simulink model "HLSDem_CalcState"  (R2016b)
settings: configuration reference "CodeGenConfigSet" (kept outside this file)
values from neighbouring files (symbols this model uses):
  EISGov_nOfsPreCtlActvFall_C = Calibration.Parameter    [init_HLSDem_CalcState.m]
  EISGov_nOfsPreCtlActvFall_CUR = Calibration.Parameter    [init_HLSDem_CalcState.m]
  EISGov_nOfsPreCtlActvFall_CURX = Calibration.Parameter    [init_HLSDem_CalcState.m]
  EISGov_nOfsPreCtlINActvFall_C = Calibration.Parameter    [init_HLSDem_CalcState.m]
  EISGov_nOfsPreCtlPrepFall_C = Calibration.Parameter    [init_HLSDem_CalcState.m]
  EISGov_nPreCtlPrepFalloffset_C = Calibration.Parameter    [init_HLSDem_CalcState.m]
  HLSDem_facGripPredef_CUR = Calibration.Parameter    [init_HLSDem_CalcState.m]
  HLSDem_facGripPredef_CURX = Calibration.Parameter    [init_HLSDem_CalcState.m]
  HLSDem_facNoGripPredef_CUR = Calibration.Parameter    [init_HLSDem_CalcState.m]
  HLSDem_facNoGripPredef_CURX = Calibration.Parameter    [init_HLSDem_CalcState.m]
  HLSDem_GripPredef_CUR = Calibration.Parameter    [init_HLSDem_CalcState.m]
  HLSDem_GripPredef_CURX = Calibration.Parameter    [init_HLSDem_CalcState.m]
  HLSDem_nOfsPredef_C = Calibration.Parameter    [init_HLSDem_CalcState.m]
  HLSDem_nOfsUndrBrk_C = Calibration.Parameter    [init_HLSDem_CalcState.m]
  HLSDem_NoGripPredef_C = Calibration.Parameter    [init_HLSDem_CalcState.m]
  HLSDem_numTempSelConv_C = Calibration.Parameter    [init_HLSDem_CalcState.m]
  HLSDem_rAPPThresFrzI_C = Calibration.Parameter    [init_HLSDem_CalcState.m]
  HLSDem_rAPPThresTrqDem_C = Calibration.Parameter    [init_HLSDem_CalcState.m]
  HLSDem_rGripUndrBrkThres_C = Calibration.Parameter    [init_HLSDem_CalcState.m]
  HLSDem_rNoGripThres_C = Calibration.Parameter    [init_HLSDem_CalcState.m]
  HLSDem_stIFrzInhib_C = Calibration.Parameter    [init_HLSDem_CalcState.m]
  HLSDem_swtAPPFrzI_C = Calibration.Parameter    [init_HLSDem_CalcState.m]
  HLSDem_swtAPPTrqDem_C = Calibration.Parameter    [init_HLSDem_CalcState.m]
  HLSDem_swtPredef_C = Calibration.Parameter    [init_HLSDem_CalcState.m]
  HLSDem_trqReqStrt_CUR = Calibration.Parameter    [init_HLSDem_CalcState.m]
  HLSDem_trqReqStrt_CURX = Calibration.Parameter    [init_HLSDem_CalcState.m]
  HLSDem_vThresUndrBrk_C = Calibration.Parameter    [init_HLSDem_CalcState.m]
  LIGov_nOffsetPreCtltrqDem_C = Calibration.Parameter    [init_HLSDem_CalcState.m]
undefined symbols (not defined in the file or in its folder): EISGov_num_conv, EngState_conv, PT_TraType_State_conv, Switch_conv
libraries: simulink x35, CXLib x2
settings Model: Creator=Administrator  LastModifiedBy=xuxingpei
settings ConfigSetRef: SourceLocation=Base Workspace

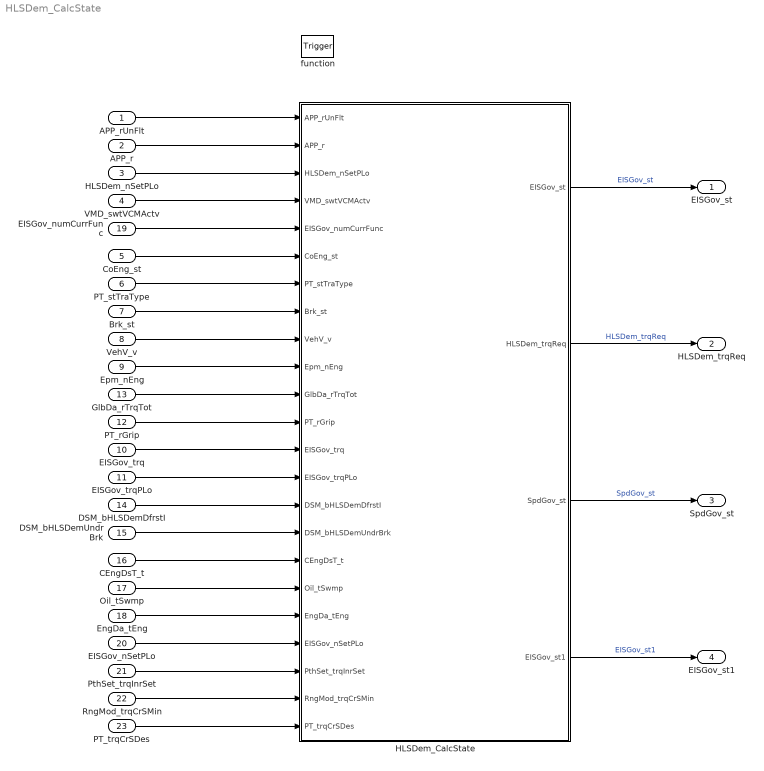
== system HLSDem_CalcState ==
  APP_rUnFlt : Inport  Tag=%  Description=Unfiltered APP value  OutMin=0  OutMax=100  OutDataTypeStr=Accpedal_rate
  APP_r : Inport  Tag=%  Description=Acceleration pedal sensor 1 value after fault handling  Port=2  OutMin=0  OutMax=100  OutDataTypeStr=Accpedal_rate
  HLSDem_nSetPLo : Inport  Tag=rpm  Description=Minimum engine speed of HLSDem  Port=3  OutMin=0  OutMax=6000  OutDataTypeStr=EngSpeed_rpm
  VMD_swtVCMActv : Inport  Description=Application parameter which Indicates whether Vehicle Control Mode(VCM) is enabled or disabled  Port=4  OutDataTypeStr=Enum: Switch_conv
  CoEng_st : Inport  Description=Engine coordinator state  Port=5  OutDataTypeStr=Enum: EngState_conv
  PT_stTraType : Inport  Description=Current transmission type  Port=6  OutDataTypeStr=Enum: PT_TraType_State_conv
  Brk_st : Inport  Description=Brake switch state  Port=7  OutMin=0  OutMax=255  OutDataTypeStr=State_uint8
  VehV_v : Inport  Tag=km/h  Description=Vehicle speed  Port=8  OutMin=0  OutMax=250  OutDataTypeStr=VehSpeed_km_h
  Epm_nEng : Inport  Tag=rpm  Description=Engine speed  Port=9  OutMin=0  OutMax=6000  OutDataTypeStr=EngSpeed_rpm
  EISGov_trq : Inport  Tag=Nm  Description=Resulted output torque of EISGov controller  Port=10  OutMin=-3276.8  OutMax=3276.7  OutDataTypeStr=Trq_Nm
  EISGov_trqPLo : Inport  Tag=Nm  Description=P-component of the lower path  Port=11  OutMin=-3276.8  OutMax=3276.7  OutDataTypeStr=Trq_Nm
  PT_rGrip : Inport  Description=Analogue value for the grip states  Port=12  OutMin=-300  OutMax=300  OutDataTypeStr=Prc_Fact100
  GlbDa_rTrqTot : Inport  Description=total ratio of the power train inclusive the differential and the converter torque ratio  Port=13  OutMin=-327  OutMax=327  OutDataTypeStr=TransRatio
  DSM_bHLSDemDfrstI : Inport  Description=Status of Fid_HLSDemDfrstI  Port=14  OutMin=0  OutMax=1  OutDataTypeStr=boolean
  DSM_bHLSDemUndrBrk : Inport  Description=Status of FId_HLSDemUndrBrk  Port=15  OutMin=0  OutMax=1  OutDataTypeStr=boolean
  CEngDsT_t : Inport  Tag=deg  Description=engine coolant temperature after filter  Port=16  OutMin=-200  OutMax=200  OutDataTypeStr=Temp_deg
  Oil_tSwmp : Inport  Tag=deg  Description=Oil temperature in oil sump  Port=17  OutMin=-50  OutMax=200  OutDataTypeStr=Temp_deg
  EngDa_tEng : Inport  Tag=deg  Description=Engine temperature  Port=18  OutMin=-1000  OutMax=1000  OutDataTypeStr=Temp_deg
  EISGov_numCurrFunc : Inport  Description=Identification name / number of the currently active EISGov client, which determines the current controller parameters  Port=19  OutDataTypeStr=Enum: EISGov_num_conv
  EISGov_nSetPLo : Inport  Tag=rpm  Description=Lower limit of the speed interval (set point speed) of the EISGov  Port=20  OutMin=0  OutMax=6000  OutDataTypeStr=EngSpeed_rpm
  PthSet_trqInrSet : Inport  Tag=Nm  Description=Inner torque set value after monitoring limitation  Port=21  OutMin=-3000  OutMax=3276.7  OutDataTypeStr=Trq_Nm
  RngMod_trqCrSMin : Inport  Tag=Nm  Description=minimal crankshaft torque  Port=22  OutMin=-3276.8  OutMax=3276.7  OutDataTypeStr=Trq_Nm
  PT_trqCrSDes : Inport  Tag=Nm  Description=Application parameter for requested propulsion torque to engine(crankshaft torque)  Port=23  OutMin=-3000  OutMax=3000  OutDataTypeStr=Trq_Nm
  function : TriggerPort  TriggerType=function-call  VariantControl=Variant
  HLSDem_CalcState : Subsystem
  EISGov_st : Outport  Description=Status information of EISGov and its clients  OutMin=0  OutMax=2147483648  OutDataTypeStr=State_uint32
  HLSDem_trqReq : Outport  Tag=Nm  Description=Requested initialisation torque to engine speed governor (with reference to the output)  Port=2  OutMin=-3000  OutMax=3000  OutDataTypeStr=Trq_Nm
  SpdGov_st : Outport  Description=status speed control SpdGov  Port=3  OutMin=0  OutMax=65535  OutDataTypeStr=State_uint16
  EISGov_st1 : Outport  Description=Status information of HLSDem client  Port=4  OutMin=0  OutMax=2147483648  OutDataTypeStr=State_uint32
  wires:
  PT_rGrip/1 -> HLSDem_CalcState/12(PT_rGrip)
  Epm_nEng/1 -> HLSDem_CalcState/10(Epm_nEng)
  APP_rUnFlt/1 -> HLSDem_CalcState/1(APP_rUnFlt)
  APP_r/1 -> HLSDem_CalcState/2(APP_r)
  VehV_v/1 -> HLSDem_CalcState/9(VehV_v)
  EISGov_numCurrFunc/1 -> HLSDem_CalcState/5(EISGov_numCurrFunc)
  PT_stTraType/1 -> HLSDem_CalcState/7(PT_stTraType)
  Brk_st/1 -> HLSDem_CalcState/8(Brk_st)
  CoEng_st/1 -> HLSDem_CalcState/6(CoEng_st)
  VMD_swtVCMActv/1 -> HLSDem_CalcState/4(VMD_swtVCMActv)
  EISGov_trq/1 -> HLSDem_CalcState/13(EISGov_trq)
  HLSDem_nSetPLo/1 -> HLSDem_CalcState/3(HLSDem_nSetPLo)
  EISGov_trqPLo/1 -> HLSDem_CalcState/14(EISGov_trqPLo)
  DSM_bHLSDemDfrstI/1 -> HLSDem_CalcState/15(DSM_bHLSDemDfrstI)
  DSM_bHLSDemUndrBrk/1 -> HLSDem_CalcState/16(DSM_bHLSDemUndrBrk)
  GlbDa_rTrqTot/1 -> HLSDem_CalcState/11(GlbDa_rTrqTot)
  HLSDem_CalcState/1(EISGov_st) -> EISGov_st/1  "EISGov_st"
  HLSDem_CalcState/2(HLSDem_trqReq) -> HLSDem_trqReq/1  "HLSDem_trqReq"
  HLSDem_CalcState/3(SpdGov_st) -> SpdGov_st/1  "SpdGov_st"
  CEngDsT_t/1 -> HLSDem_CalcState/17(CEngDsT_t)
  Oil_tSwmp/1 -> HLSDem_CalcState/18(Oil_tSwmp)
  EngDa_tEng/1 -> HLSDem_CalcState/19(EngDa_tEng)
  HLSDem_CalcState/4(EISGov_st1) -> EISGov_st1/1  "EISGov_st1"
  EISGov_nSetPLo/1 -> HLSDem_CalcState/20(EISGov_nSetPLo)
  PthSet_trqInrSet/1 -> HLSDem_CalcState/21(PthSet_trqInrSet)
  RngMod_trqCrSMin/1 -> HLSDem_CalcState/22(RngMod_trqCrSMin)
  PT_trqCrSDes/1 -> HLSDem_CalcState/23(PT_trqCrSDes)

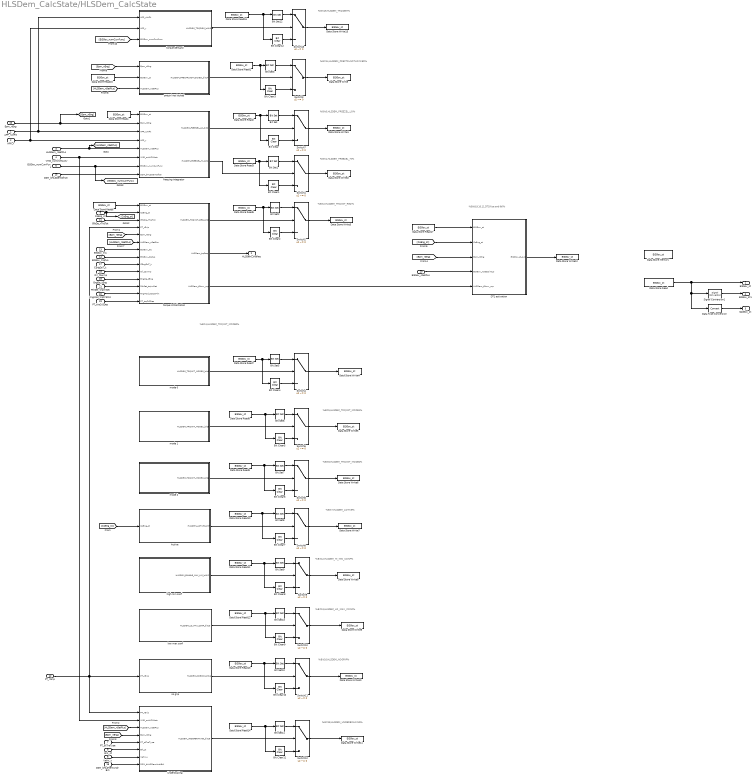
== system HLSDem_CalcState/HLSDem_CalcState ==
  note: %Bit4,HLSDEM_TRQINIT_MODE0%
  note: %Bit14,HLSDEM_PRECTRLNOTLOCKED%
  note: %Bit0,HLSDEM_FREEZEL_LO%
  note: %Bit1,HLSDEM_FREEZEL_HI%
  note: %Bit2,HLSDEM_TRQINIT_REQ%
  note: %Bit5,HLSDEM_TRQINIT_MODE1%
  note: %Bit6,HLSDEM_TRQINIT_MODE2%
  note: %Bit7,HLSDEM_ACTIVE%
  note: %Bit13,HLSDEM_LO_MAX_CONF%
  note: %Bit12,HLSDEM_HI_MIN_CONF%
  note: %Bit16,HLSDEM_NOGRIP%
  note: %Bit18,HLSDEM_UNDERBRAKING%
  note: %Bit19,HLSDEM_TRQDEM%
  note: %Bit8,9,10,11,DT1Rise and fall%
  APP_rUnFlt : Inport
  APP_r : Inport  Port=2
  HLSDem_nSetPLo : Inport  Port=3
  VMD_swtVCMActv : Inport  Port=4
  EISGov_numCurrFunc : Inport  Port=5
  CoEng_st : Inport  Port=6
  PT_stTraType : Inport  Port=7
  Brk_st : Inport  Port=8
  VehV_v : Inport  Port=9
  Epm_nEng : Inport  Port=10
  GlbDa_rTrqTot : Inport  Port=11
  PT_rGrip : Inport  Port=12
  EISGov_trq : Inport  Port=13
  EISGov_trqPLo : Inport  Port=14
  DSM_bHLSDemDfrstI : Inport  Port=15
  DSM_bHLSDemUndrBrk : Inport  Port=16
  CEngDsT_t : Inport  Tag=deg  Description=engine coolant temperature after filter  Port=17  OutMin=-200  OutMax=200  OutDataTypeStr=Temp_deg
  Oil_tSwmp : Inport  Tag=deg  Description=Oil temperature in oil sump  Port=18  OutMin=-50  OutMax=200  OutDataTypeStr=Temp_deg
  EngDa_tEng : Inport  Tag=deg  Description=Engine temperature  Port=19  OutMin=-1000  OutMax=1000  OutDataTypeStr=Temp_deg
  EISGov_nSetPLo : Inport  Tag=rpm  Description=Lower limit of the speed interval (set point speed) of the EISGov  Port=20  OutMin=0  OutMax=6000  OutDataTypeStr=EngSpeed_rpm
  PthSet_trqInrSet : Inport  Tag=Nm  Description=Inner torque set value after monitoring limitation  Port=21  OutMin=-3000  OutMax=3276.7  OutDataTypeStr=Trq_Nm
  RngMod_trqCrSMin : Inport  Port=22
  PT_trqCrSDes : Inport  Port=23
  Active : Subsystem
  Bit Clear : simulink/Logic and Bit Operations/Bit Clear  iBit=0
  Bit Clear1 : simulink/Logic and Bit Operations/Bit Clear  iBit=1
  Bit Clear10 : simulink/Logic and Bit Operations/Bit Clear  iBit=16
  Bit Clear11 : simulink/Logic and Bit Operations/Bit Clear  iBit=18
  Bit Clear12 : simulink/Logic and Bit Operations/Bit Clear  iBit=19
  Bit Clear2 : simulink/Logic and Bit Operations/Bit Clear  iBit=2
  Bit Clear3 : simulink/Logic and Bit Operations/Bit Clear  iBit=14
  Bit Clear4 : simulink/Logic and Bit Operations/Bit Clear  iBit=4
  Bit Clear5 : simulink/Logic and Bit Operations/Bit Clear  iBit=5
  Bit Clear6 : simulink/Logic and Bit Operations/Bit Clear  iBit=6
  Bit Clear7 : simulink/Logic and Bit Operations/Bit Clear  iBit=7
  Bit Clear8 : simulink/Logic and Bit Operations/Bit Clear  iBit=12
  Bit Clear9 : simulink/Logic and Bit Operations/Bit Clear  iBit=13
  Bit Set : simulink/Logic and Bit Operations/Bit Set  iBit=0
  Bit Set1 : simulink/Logic and Bit Operations/Bit Set  iBit=1
  Bit Set10 : simulink/Logic and Bit Operations/Bit Set  iBit=16
  Bit Set11 : simulink/Logic and Bit Operations/Bit Set  iBit=18
  Bit Set12 : simulink/Logic and Bit Operations/Bit Set  iBit=19
  Bit Set13 : simulink/Logic and Bit Operations/Bit Set  iBit=13
  Bit Set2 : simulink/Logic and Bit Operations/Bit Set  iBit=2
  Bit Set3 : simulink/Logic and Bit Operations/Bit Set  iBit=14
  Bit Set5 : simulink/Logic and Bit Operations/Bit Set  iBit=4
  Bit Set6 : simulink/Logic and Bit Operations/Bit Set  iBit=5
  Bit Set7 : simulink/Logic and Bit Operations/Bit Set  iBit=6
  Bit Set8 : simulink/Logic and Bit Operations/Bit Set  iBit=7
  Bit Set9 : simulink/Logic and Bit Operations/Bit Set  iBit=12
  DT1 activation : Subsystem
  Data Store Memory : DataStoreMemory  DataStoreName=EISGov_st  ReadBeforeWriteMsg=warning  WriteAfterWriteMsg=warning  WriteAfterReadMsg=warning  ShowAdditionalParam=off
  Data Store Read{,1..17} (18 alike) : DataStoreRead  DataStoreName=EISGov_st
  Data Store Write{,1..13} (14 alike) : DataStoreWrite  DataStoreName=EISGov_st
  Data Type Conversion : DataTypeConversion
  Signal Conversion1 : SignalConversion  OverrideOpt=off
  Switch{1..13} (13 alike) : Switch  Criteria=u2 ~= 0
  Underbraking : Subsystem
  freezing integrator : Subsystem
  high min conf : Subsystem
  low max conf : Subsystem
  mode 0 : Subsystem
  mode 1 : Subsystem
  mode 2 : Subsystem
  no grip : Subsystem
  prectrl not locked : Subsystem
  torque demand : Subsystem
  torque initialization : Subsystem  Priority=2
  EISGov_st : Outport
  HLSDem_trqReq : Outport  Port=2
  SpdGov_st : Outport  Port=3
  EISGov_st1 : Outport  Port=4
  wires:
  HLSDem_nSetPLo/1 -> freezing integrator/5(HLSDem_nSetPLo), [HLSDem_nSetPLo]
  PT_rGrip/1 -> Underbraking/1(PT_rGrip), no grip/1(PT_rGrip), torque initialization/4(PT_rGrip)
  APP_r/1 -> torque demand/2(APP_r), freezing integrator/4(APP_r)
  EISGov_trq/1 -> torque initialization/7(EISGov_trq)
  Data Store Read4/1 -> freezing integrator/1(EISGov_st)
  APP_rUnFlt/1 -> torque demand/1(APP_rUnFlt), freezing integrator/3(APP_rUnFlt)
  CoEng_st/1 -> [CoEng_st], torque initialization/2(CoEng_st)
  VMD_swtVCMActv/1 -> Underbraking/2("VMD_swtVCMActv "), freezing integrator/6(VMD_swtVCMActv)
  GlbDa_rTrqTot/1 -> torque initialization/3(GlbDa_rTrqTot)
  EISGov_trqPLo/1 -> torque initialization/8(EISGov_trqPLo)
  Epm_nEng/1 -> freezing integrator/2(Epm_nEng), [Epm_nEng]
  [Epm_nEng] -> torque initialization/5(Epm_nEng)
  PT_stTraType/1 -> Underbraking/5(PT_stTraType)
  EISGov_numCurrFunc/1 -> [EISGov_numCurrFunc], freezing integrator/7(EISGov_numCurrFunc)
  [Epm_nEng] -> Underbraking/4(Epm_nEng)
  [HLSDem_nSetPLo] -> Underbraking/3(HLSDem_nSetPLo)
  [HLSDem_nSetPLo] -> torque initialization/6(HLSDem_nSetPLo)
  torque initialization/2(HLSDem_trqReq) -> HLSDem_trqReq/1
  DSM_bHLSDemDfrstI/1 -> freezing integrator/8(DSM_bHLSDemDfrstI)
  Brk_st/1 -> Underbraking/6(Brk_st)
  VehV_v/1 -> Underbraking/7(VehV_v)
  DSM_bHLSDemUndrBrk/1 -> Underbraking/8(DSM_bHLSDemUndrBrk)
  Data Store Read6/1 -> torque initialization/1(EISGov_st)
  Data Store Read/1 -> Data Type Conversion/1, Signal Conversion1/1, EISGov_st/1
  CEngDsT_t/1 -> torque initialization/9(CEngDsT_t)
  Oil_tSwmp/1 -> torque initialization/10(Oil_tSwmp)
  EngDa_tEng/1 -> torque initialization/11(EngDa_tEng)
  Data Type Conversion/1 -> SpdGov_st/1
  Data Store Read15/1 -> prectrl not locked/2(EISGov_st)
  Switch3/1 -> Data Store Write/1
  Data Store Read1/1 -> Bit Set3/1, Bit Clear3/1
  [Epm_nEng] -> prectrl not locked/1(Epm_nEng)
  [HLSDem_nSetPLo] -> prectrl not locked/3(HLSDem_nSetPLo)
  prectrl not locked/1(HLSDEM_PRECTRLNOTLOCKED_bit14) -> Switch3/2
  Bit Set3/1 -> Switch3/1
  Bit Clear3/1 -> Switch3/3
  Switch1/1 -> Data Store Write2/1
  Data Store Read3/1 -> Bit Set1/1, Bit Clear1/1
  Switch7/1 -> Data Store Write1/1
  Data Store Read2/1 -> Bit Set/1, Bit Clear/1
  freezing integrator/1(HLSDEM_FREEZEL_LO_bit0) -> Switch7/2
  Bit Set/1 -> Switch7/1
  Bit Clear/1 -> Switch7/3
  freezing integrator/2(HLSDEM_FREEZEL_HI_bit1) -> Switch1/2
  Bit Set1/1 -> Switch1/1
  Bit Clear1/1 -> Switch1/3
  Switch2/1 -> Data Store Write3/1
  Data Store Read5/1 -> Bit Set2/1, Bit Clear2/1
  torque initialization/1(HLSDEM_TRQINIT_REQ_bit2) -> Switch2/2
  Bit Set2/1 -> Switch2/1
  Bit Clear2/1 -> Switch2/3
  Switch10/1 -> Data Store Write9/1
  Data Store Read12/1 -> Bit Set13/1, Bit Clear9/1
  Switch9/1 -> Data Store Write8/1
  Data Store Read11/1 -> Bit Set9/1, Bit Clear8/1
  Switch8/1 -> Data Store Write7/1
  Data Store Read10/1 -> Bit Set8/1, Bit Clear7/1
  Switch6/1 -> Data Store Write6/1
  Data Store Read9/1 -> Bit Set7/1, Bit Clear6/1
  Switch5/1 -> Data Store Write5/1
  Data Store Read8/1 -> Bit Set6/1, Bit Clear5/1
  Switch4/1 -> Data Store Write4/1
  Data Store Read7/1 -> Bit Set5/1, Bit Clear4/1
  [CoEng_st] -> Active/1(CoEng_st)
  mode 0/1(HLSDEM_TRQINIT_MODE0_bit4) -> Switch4/2
  Bit Set5/1 -> Switch4/1
  Bit Clear4/1 -> Switch4/3
  mode 1/1(HLSDEM_TRQINIT_MODE1_bit5) -> Switch5/2
  Bit Set6/1 -> Switch5/1
  Bit Clear5/1 -> Switch5/3
  mode 2/1(HLSDEM_TRQINIT_MODE2_bit6) -> Switch6/2
  Bit Set7/1 -> Switch6/1
  Bit Clear6/1 -> Switch6/3
  Active/1(HLSDEM_ACTIVE_bit7) -> Switch8/2
  Bit Set8/1 -> Switch8/1
  Bit Clear7/1 -> Switch8/3
  high min conf/1(HLSDEM_ENABLE_MAX_LIM_bit12) -> Switch9/2
  Bit Set9/1 -> Switch9/1
  Bit Clear8/1 -> Switch9/3
  low max conf/1(HLSDEM_LO_MAX_CONF_bit13) -> Switch10/2
  Bit Set13/1 -> Switch10/1
  Bit Clear9/1 -> Switch10/3
  Switch13/1 -> Data Store Write13/1
  Data Store Read16/1 -> Bit Set12/1, Bit Clear12/1
  Switch12/1 -> Data Store Write11/1
  Data Store Read14/1 -> Bit Set11/1, Bit Clear11/1
  Switch11/1 -> Data Store Write10/1
  Data Store Read13/1 -> Bit Set10/1, Bit Clear10/1
  no grip/1(HLSDEM_NOGRIP_bit16) -> Switch11/2
  Bit Set10/1 -> Switch11/1
  Bit Clear10/1 -> Switch11/3
  Underbraking/1(HLSDEM_UNDERBRAKING_bit18) -> Switch12/2
  Bit Set11/1 -> Switch12/1
  Bit Clear11/1 -> Switch12/3
  torque demand/1(HLSDEM_TRQDEM_bit19) -> Switch13/2
  Bit Set12/1 -> Switch13/1
  Bit Clear12/1 -> Switch13/3
  Signal Conversion1/1 -> EISGov_st1/1
  [CoEng_st] -> DT1 activation/2(CoEng_st)
  EISGov_nSetPLo/1 -> DT1 activation/4(EISGov_nSetpointLo)
  [Epm_nEng] -> DT1 activation/3(Epm_nEng)
  DT1 activation/1(EISGov_st_out) -> Data Store Write12/1
  Data Store Read17/1 -> DT1 activation/1(EISGov_st)
  [EISGov_numCurrFunc] -> torque demand/3(EISGov_numCurrFunc)
  PthSet_trqInrSet/1 -> torque initialization/12(PthSet_trqInrSet)
  RngMod_trqCrSMin/1 -> torque initialization/13(RngMod_trqCrSMin)
  PT_trqCrSDes/1 -> torque initialization/14(PT_trqCrSDes)
  torque initialization/3(HLSDem_tConv_mp) -> DT1 activation/5(HLSDem_tConv_mp)

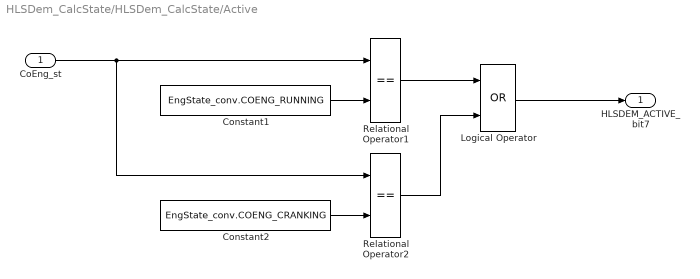
== system HLSDem_CalcState/HLSDem_CalcState/Active ==
  CoEng_st : Inport
  Constant1 : Constant  Value=EngState_conv.COENG_RUNNING  OutDataTypeStr=Inherit: Inherit via back propagation
  Constant2 : Constant  Value=EngState_conv.COENG_CRANKING  OutDataTypeStr=Inherit: Inherit via back propagation
  Logical Operator : Logic  Operator=OR  AllPortsSameDT=off  OutDataTypeStr=boolean
  Relational Operator1 : RelationalOperator  Operator===  OutDataTypeStr=boolean  RndMeth=Nearest  InputSameDT=on
  Relational Operator2 : RelationalOperator  Operator===  OutDataTypeStr=boolean  RndMeth=Nearest  InputSameDT=on
  HLSDEM_ACTIVE_bit7 : Outport
  wires:
  CoEng_st/1 -> Relational Operator2/1, Relational Operator1/1
  Constant1/1 -> Relational Operator1/2
  Logical Operator/1 -> HLSDEM_ACTIVE_bit7/1
  Relational Operator1/1 -> Logical Operator/1
  Constant2/1 -> Relational Operator2/2
  Relational Operator2/1 -> Logical Operator/2

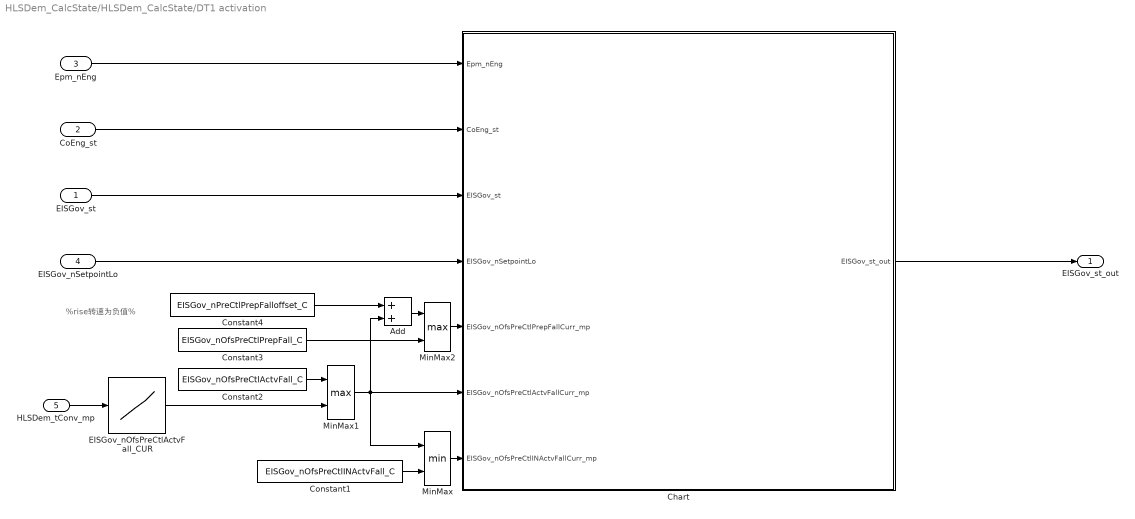
== system HLSDem_CalcState/HLSDem_CalcState/DT1 activation ==
  note: %rise转速为负值%
  EISGov_st : Inport  OutDataTypeStr=State_uint32
  CoEng_st : Inport  Port=2
  Epm_nEng : Inport  Port=3
  EISGov_nSetpointLo : Inport  Port=4
  HLSDem_tConv_mp : Inport  Port=5
  Add : Sum  SaturateOnIntegerOverflow=on
  Chart : Stateflow chart  TreatAsAtomicUnit=on
  Constant1 : Constant  Value=EISGov_nOfsPreCtlINActvFall_C
  Constant2 : Constant  Value=EISGov_nOfsPreCtlActvFall_C
  Constant3 : Constant  Value=EISGov_nOfsPreCtlPrepFall_C
  Constant4 : Constant  Value=EISGov_nPreCtlPrepFalloffset_C
  EISGov_nOfsPreCtlActvFall_CUR : Lookup_n-D  NumberOfTableDimensions=1  BreakpointsForDimension1=EISGov_nOfsPreCtlActvFall_CURX  Table=EISGov_nOfsPreCtlActvFall_CUR  ExtrapMethod=Clip  InternalRulePriority=Speed  OutDataTypeStr=Inherit: Inherit via back propagation  RndMeth=Simplest  SaturateOnIntegerOverflow=on
  MinMax : MinMax  Inputs=2
  MinMax1 : MinMax  Function=max  Inputs=2
  MinMax2 : MinMax  Function=max  Inputs=2
  EISGov_st_out : Outport
  wires:
  EISGov_st/1 -> Chart/3(EISGov_st)
  EISGov_nSetpointLo/1 -> Chart/4(EISGov_nSetpointLo)
  CoEng_st/1 -> Chart/2(CoEng_st)
  Epm_nEng/1 -> Chart/1(Epm_nEng)
  Chart/1(EISGov_st_out) -> EISGov_st_out/1
  MinMax/1 -> Chart/7(EISGov_nOfsPreCtlINActvFallCurr_mp)
  Constant1/1 -> MinMax/2
  HLSDem_tConv_mp/1 -> EISGov_nOfsPreCtlActvFall_CUR/1
  Constant2/1 -> MinMax1/1
  EISGov_nOfsPreCtlActvFall_CUR/1 -> MinMax1/2
  MinMax1/1 -> MinMax/1, Add/2, Chart/6(EISGov_nOfsPreCtlActvFallCurr_mp)
  Constant3/1 -> MinMax2/2
  MinMax2/1 -> Chart/5(EISGov_nOfsPreCtlPrepFallCurr_mp)
  Add/1 -> MinMax2/1
  Constant4/1 -> Add/1

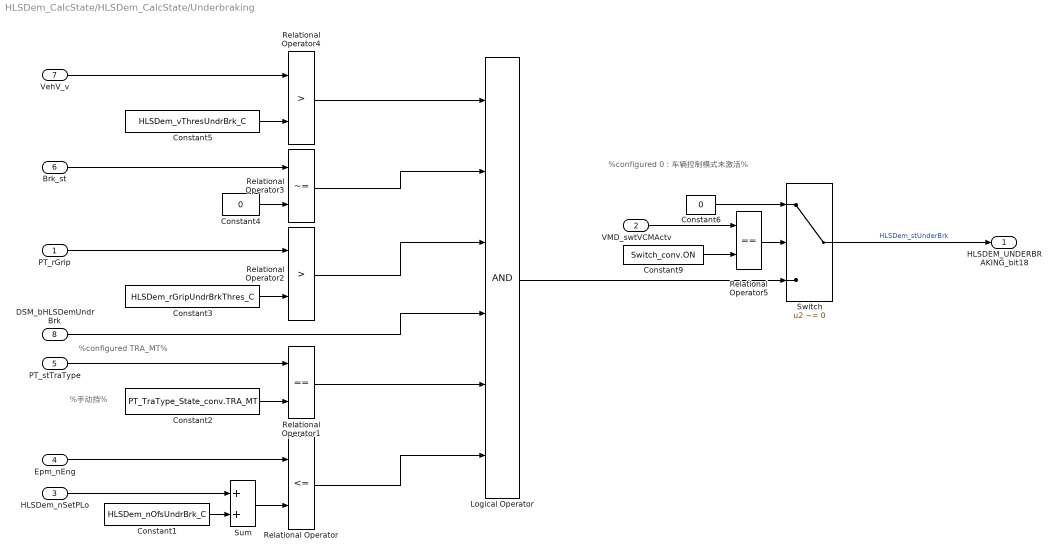
== system HLSDem_CalcState/HLSDem_CalcState/Underbraking ==
  note: %手动挡%
  note: %configured 0：车辆控制模式未激活%
  note: %configured TRA_MT%
  PT_rGrip : Inport
  "VMD_swtVCMActv " : Inport  Port=2
  HLSDem_nSetPLo : Inport  Port=3
  Epm_nEng : Inport  Port=4
  PT_stTraType : Inport  Port=5
  Brk_st : Inport  Port=6
  VehV_v : Inport  Port=7
  DSM_bHLSDemUndrBrk : Inport  Port=8
  Constant1 : Constant  Value=HLSDem_nOfsUndrBrk_C
  Constant2 : Constant  Value=PT_TraType_State_conv.TRA_MT  OutDataTypeStr=Inherit: Inherit via back propagation
  Constant3 : Constant  Value=HLSDem_rGripUndrBrkThres_C
  Constant4 : Constant  Value=0  OutDataTypeStr=Inherit: Inherit via back propagation
  Constant5 : Constant  Value=HLSDem_vThresUndrBrk_C
  Constant6 : Constant  Value=0  OutDataTypeStr=Inherit: Inherit via back propagation
  Constant9 : Constant  Value=Switch_conv.ON  OutDataTypeStr=Enum:Switch_conv
  Logical Operator : Logic  Inputs=6  OutDataTypeStr=boolean
  Relational Operator : RelationalOperator  Operator=<=  OutDataTypeStr=boolean  RndMeth=Simplest  InputSameDT=on
  Relational Operator1 : RelationalOperator  Operator===  OutDataTypeStr=boolean  RndMeth=Simplest  InputSameDT=on
  Relational Operator2 : RelationalOperator  Operator=>  OutDataTypeStr=boolean  RndMeth=Simplest  InputSameDT=on
  Relational Operator3 : RelationalOperator  Operator=~=  OutDataTypeStr=boolean  RndMeth=Simplest  InputSameDT=on
  Relational Operator4 : RelationalOperator  Operator=>  OutDataTypeStr=boolean  RndMeth=Simplest  InputSameDT=on
  Relational Operator5 : RelationalOperator  Operator===  OutDataTypeStr=boolean  RndMeth=Nearest  InputSameDT=on
  Sum : Sum  SaturateOnIntegerOverflow=on  InputSameDT=on
  Switch : Switch  Criteria=u2 ~= 0  InputSameDT=on
  HLSDEM_UNDERBRAKING_bit18 : Outport
  wires:
  Relational Operator5/1 -> Switch/2
  Constant4/1 -> Relational Operator3/2
  Constant3/1 -> Relational Operator2/2
  PT_rGrip/1 -> Relational Operator2/1
  Logical Operator/1 -> Switch/3
  Relational Operator2/1 -> Logical Operator/3
  Brk_st/1 -> Relational Operator3/1
  VehV_v/1 -> Relational Operator4/1
  Relational Operator3/1 -> Logical Operator/2
  Sum/1 -> Relational Operator/2
  Constant5/1 -> Relational Operator4/2
  Relational Operator4/1 -> Logical Operator/1
  "VMD_swtVCMActv "/1 -> Relational Operator5/1
  Constant9/1 -> Relational Operator5/2
  Epm_nEng/1 -> Relational Operator/1
  HLSDem_nSetPLo/1 -> Sum/1
  Switch/1 -> HLSDEM_UNDERBRAKING_bit18/1  "HLSDem_stUnderBrk"
  Constant6/1 -> Switch/1
  DSM_bHLSDemUndrBrk/1 -> Logical Operator/4
  Relational Operator1/1 -> Logical Operator/5
  Relational Operator/1 -> Logical Operator/6
  Constant1/1 -> Sum/2
  Constant2/1 -> Relational Operator1/2
  PT_stTraType/1 -> Relational Operator1/1

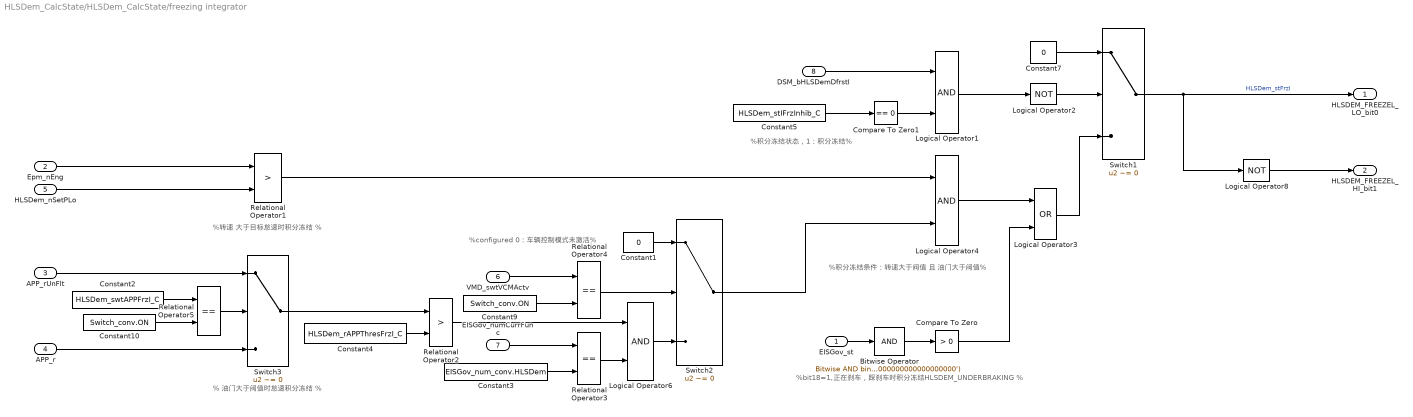
== system HLSDem_CalcState/HLSDem_CalcState/freezing integrator ==
  note: %积分冻结条件：转速大于阀值 且 油门大于阀值%
  note: %积分冻结状态，1：积分冻结%
  note: % 油门大于阀值时怠速积分冻结 %
  note: %bit18=1,正在刹车，踩刹车时积分冻结HLSDEM_UNDERBRAKING %
  note: %configured 0：车辆控制模式未激活%
  note: %转速 大于目标怠速时积分冻结 %
  EISGov_st : Inport
  Epm_nEng : Inport  Port=2
  APP_rUnFlt : Inport  Port=3
  APP_r : Inport  Port=4
  HLSDem_nSetPLo : Inport  Port=5
  VMD_swtVCMActv : Inport  Port=6
  EISGov_numCurrFunc : Inport  Port=7
  DSM_bHLSDemDfrstI : Inport  Port=8
  Bitwise Operator : simulink/Logic and Bit Operations/Bitwise Operator  logicop=AND  UseBitMask=on  BitMask=bin2dec('00000000000001000000000000000000')  BitMaskRealWorld=Stored Integer
  Compare To Zero : simulink/Logic and Bit Operations/Compare To Zero  relop=>  OutDataTypeStr=boolean
  Compare To Zero1 : simulink/Logic and Bit Operations/Compare To Zero  relop===  OutDataTypeStr=boolean
  Constant1 : Constant  Value=0  OutDataTypeStr=Inherit: Inherit via back propagation
  Constant10 : Constant  Value=Switch_conv.ON  OutDataTypeStr=Enum:Switch_conv
  Constant2 : Constant  Value=HLSDem_swtAPPFrzI_C
  Constant3 : Constant  Value=EISGov_num_conv.HLSDem
  Constant4 : Constant  Value=HLSDem_rAPPThresFrzI_C
  Constant5 : Constant  Value=HLSDem_stIFrzInhib_C
  Constant7 : Constant  Value=0  OutDataTypeStr=boolean
  Constant9 : Constant  Value=Switch_conv.ON  OutDataTypeStr=Enum:Switch_conv
  Logical Operator1 : Logic  OutDataTypeStr=boolean
  Logical Operator2 : Logic  Operator=NOT  AllPortsSameDT=off  OutDataTypeStr=boolean
  Logical Operator3 : Logic  Operator=OR  OutDataTypeStr=boolean
  Logical Operator4 : Logic  OutDataTypeStr=boolean
  Logical Operator6 : Logic  OutDataTypeStr=boolean
  Logical Operator8 : Logic  Operator=NOT  AllPortsSameDT=off  OutDataTypeStr=boolean
  Relational Operator1 : RelationalOperator  Operator=>  OutDataTypeStr=boolean  RndMeth=Nearest  InputSameDT=on
  Relational Operator2 : RelationalOperator  Operator=>  OutDataTypeStr=boolean  RndMeth=Nearest  InputSameDT=on
  Relational Operator3 : RelationalOperator  Operator===  OutDataTypeStr=boolean  RndMeth=Nearest  InputSameDT=on
  Relational Operator4 : RelationalOperator  Operator===  OutDataTypeStr=boolean  RndMeth=Nearest  InputSameDT=on
  Relational Operator5 : RelationalOperator  Operator===  OutDataTypeStr=boolean  RndMeth=Nearest  InputSameDT=on
  Switch1 : Switch  Criteria=u2 ~= 0  InputSameDT=on
  Switch2 : Switch  Criteria=u2 ~= 0  InputSameDT=on
  Switch3 : Switch  Criteria=u2 ~= 0  InputSameDT=on
  HLSDEM_FREEZEL_LO_bit0 : Outport
  HLSDEM_FREEZEL_HI_bit1 : Outport  Port=2
  wires:
  EISGov_numCurrFunc/1 -> Relational Operator3/1
  VMD_swtVCMActv/1 -> Relational Operator4/1
  Logical Operator1/1 -> Logical Operator2/1
  Constant9/1 -> Relational Operator4/2
  Constant3/1 -> Relational Operator3/2
  Relational Operator3/1 -> Logical Operator6/2
  Relational Operator4/1 -> Switch2/2
  Constant10/1 -> Relational Operator5/2
  Relational Operator5/1 -> Switch3/2
  Switch3/1 -> Relational Operator2/1
  APP_r/1 -> Switch3/3
  Constant1/1 -> Switch2/1
  HLSDem_nSetPLo/1 -> Relational Operator1/2
  Relational Operator2/1 -> Logical Operator6/1
  APP_rUnFlt/1 -> Switch3/1
  Constant2/1 -> Relational Operator5/1
  Logical Operator6/1 -> Switch2/3
  Epm_nEng/1 -> Relational Operator1/1
  Constant4/1 -> Relational Operator2/2
  Switch1/1 -> HLSDEM_FREEZEL_LO_bit0/1, Logical Operator8/1  "HLSDem_stFrzI"
  Constant7/1 -> Switch1/1
  Logical Operator3/1 -> Switch1/3
  Bitwise Operator/1 -> Compare To Zero/1
  Logical Operator2/1 -> Switch1/2
  Logical Operator8/1 -> HLSDEM_FREEZEL_HI_bit1/1
  Compare To Zero/1 -> Logical Operator3/2
  Constant5/1 -> Compare To Zero1/1
  Relational Operator1/1 -> Logical Operator4/1
  Compare To Zero1/1 -> Logical Operator1/2
  Switch2/1 -> Logical Operator4/2
  EISGov_st/1 -> Bitwise Operator/1
  DSM_bHLSDemDfrstI/1 -> Logical Operator1/1
  Logical Operator4/1 -> Logical Operator3/1

== system HLSDem_CalcState/HLSDem_CalcState/high min conf ==
  note: %Enable the EISGov MAX-limitation EISGov_st[1].14 = 1 %
  Constant7 : Constant  OutDataTypeStr=boolean
  HLSDEM_ENABLE_MAX_LIM_bit12 : Outport
  wires:
  Constant7/1 -> HLSDEM_ENABLE_MAX_LIM_bit12/1

== system HLSDem_CalcState/HLSDem_CalcState/low max conf ==
  note: %MAX-configuration of lower EISGov PI-path EISGov_st[1].13 = 1 %
  Constant7 : Constant  OutDataTypeStr=boolean
  HLSDEM_LO_MAX_CONF_bit13 : Outport
  wires:
  Constant7/1 -> HLSDEM_LO_MAX_CONF_bit13/1

== system HLSDem_CalcState/HLSDem_CalcState/mode 0 ==
  note: %bit 5,bit 4
      | 0,0=绝对赋值：EISGov_trq(k)=EISGov_trqReq(k);
      | 0,1=相对赋值：EISGov_trq(k) = EISGov_trq(k-1) + EISGov_trqReq(k)；
      | 1,0=最大赋值： EISGov_trq(k) = max( EISGov_trq(k-1), EISGov_trqReq(k) )；
      | 1,1= 最小赋值： EISGov_trq(k) = min( EISGov_trq(k-1), EISGov_trqReq(k) ) ；
      | %
  Constant3 : Constant  Value=0  OutDataTypeStr=boolean
  HLSDEM_TRQINIT_MODE0_bit4 : Outport
  wires:
  Constant3/1 -> HLSDEM_TRQINIT_MODE0_bit4/1

== system HLSDem_CalcState/HLSDem_CalcState/mode 1 ==
  note: %bit 5,bit 4
      | 0,0=绝对赋值：EISGov_trq(k)=EISGov_trqReq(k);
      | 0,1=相对赋值：EISGov_trq(k) = EISGov_trq(k-1) + EISGov_trqReq(k)；
      | 1,0=最大赋值： EISGov_trq(k) = max( EISGov_trq(k-1), EISGov_trqReq(k) )；
      | 1,1= 最小赋值： EISGov_trq(k) = min( EISGov_trq(k-1), EISGov_trqReq(k) ) ；
      | %
  Constant3 : Constant  Value=0  OutDataTypeStr=boolean
  HLSDEM_TRQINIT_MODE1_bit5 : Outport
  wires:
  Constant3/1 -> HLSDEM_TRQINIT_MODE1_bit5/1

== system HLSDem_CalcState/HLSDem_CalcState/mode 2 ==
  note: %single/multiple initialization demand (0/1) %
  Constant3 : Constant  Value=0  OutDataTypeStr=boolean
  HLSDEM_TRQINIT_MODE2_bit6 : Outport
  wires:
  Constant3/1 -> HLSDEM_TRQINIT_MODE2_bit6/1

== system HLSDem_CalcState/HLSDem_CalcState/no grip ==
  PT_rGrip : Inport
  Constant3 : Constant  Value=HLSDem_rNoGripThres_C
  Relational Operator3 : RelationalOperator  Operator=<  OutDataTypeStr=boolean  RndMeth=Nearest  InputSameDT=on
  HLSDEM_NOGRIP_bit16 : Outport
  wires:
  Constant3/1 -> Relational Operator3/2
  Relational Operator3/1 -> HLSDEM_NOGRIP_bit16/1
  PT_rGrip/1 -> Relational Operator3/1

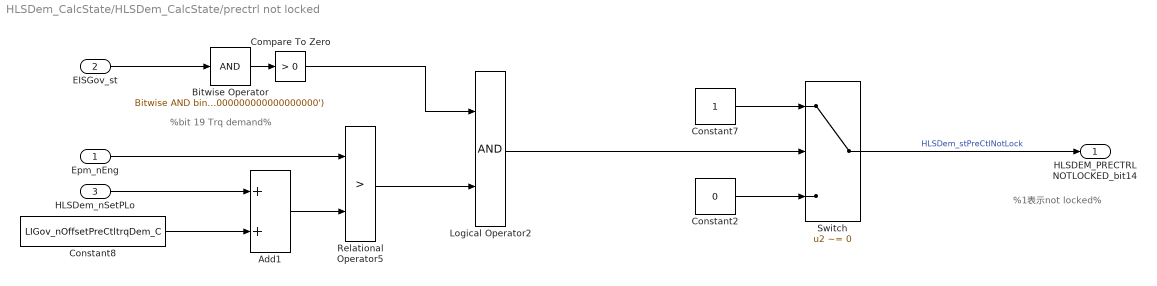
== system HLSDem_CalcState/HLSDem_CalcState/prectrl not locked ==
  note: %bit 19 Trq demand%
  note: %1表示not locked%
  Epm_nEng : Inport
  EISGov_st : Inport  Port=2
  HLSDem_nSetPLo : Inport  Port=3
  Add1 : Sum
  Bitwise Operator : simulink/Logic and Bit Operations/Bitwise Operator  logicop=AND  UseBitMask=on  BitMask=bin2dec('00000000000010000000000000000000')  BitMaskRealWorld=Stored Integer
  Compare To Zero : simulink/Logic and Bit Operations/Compare To Zero  relop=>  OutDataTypeStr=boolean
  Constant2 : Constant  Value=0  OutDataTypeStr=boolean
  Constant7 : Constant  OutDataTypeStr=boolean
  Constant8 : Constant  Value=LIGov_nOffsetPreCtltrqDem_C
  Logical Operator2 : Logic  OutDataTypeStr=boolean
  Relational Operator5 : RelationalOperator  Operator=>  OutDataTypeStr=boolean  RndMeth=Nearest  InputSameDT=on
  Switch : Switch  Criteria=u2 ~= 0  InputSameDT=on
  HLSDEM_PRECTRLNOTLOCKED_bit14 : Outport
  wires:
  Constant2/1 -> Switch/3
  Constant7/1 -> Switch/1
  Switch/1 -> HLSDEM_PRECTRLNOTLOCKED_bit14/1  "HLSDem_stPreCtlNotLock"
  Logical Operator2/1 -> Switch/2
  Compare To Zero/1 -> Logical Operator2/1
  Relational Operator5/1 -> Logical Operator2/2
  Constant8/1 -> Add1/2
  HLSDem_nSetPLo/1 -> Add1/1
  Add1/1 -> Relational Operator5/2
  Epm_nEng/1 -> Relational Operator5/1
  EISGov_st/1 -> Bitwise Operator/1
  Bitwise Operator/1 -> Compare To Zero/1

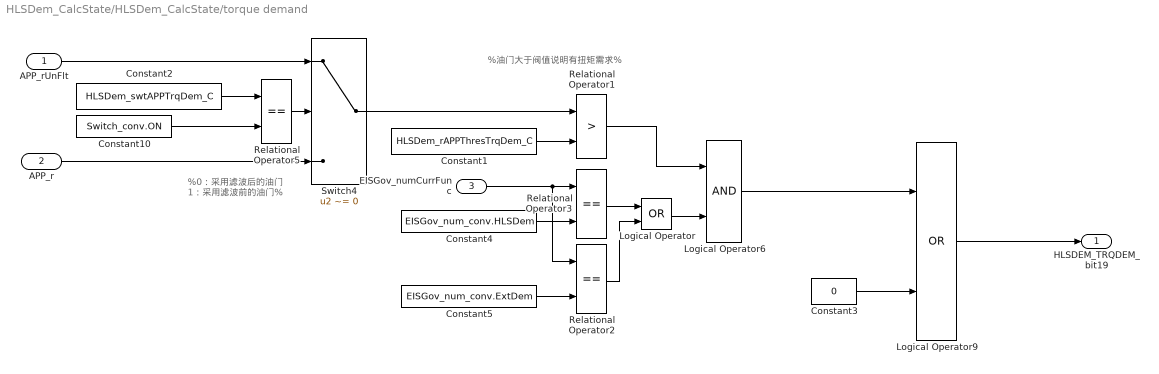
== system HLSDem_CalcState/HLSDem_CalcState/torque demand ==
  note: %0：采用滤波后的油门
      | 1：采用滤波前的油门%
  note: %油门大于阀值说明有扭矩需求%
  APP_rUnFlt : Inport
  APP_r : Inport  Port=2
  EISGov_numCurrFunc : Inport  Port=3
  Constant1 : Constant  Value=HLSDem_rAPPThresTrqDem_C
  Constant10 : Constant  Value=Switch_conv.ON  OutDataTypeStr=Enum:Switch_conv
  Constant2 : Constant  Value=HLSDem_swtAPPTrqDem_C
  Constant3 : Constant  Value=0  OutDataTypeStr=Inherit: Inherit via back propagation
  Constant4 : Constant  Value=EISGov_num_conv.HLSDem
  Constant5 : Constant  Value=EISGov_num_conv.ExtDem
  Logical Operator : Logic  Operator=OR  AllPortsSameDT=off  OutDataTypeStr=boolean
  Logical Operator6 : Logic  OutDataTypeStr=boolean
  Logical Operator9 : Logic  Operator=OR  OutDataTypeStr=boolean
  Relational Operator1 : RelationalOperator  Operator=>  OutDataTypeStr=boolean  RndMeth=Nearest  InputSameDT=on
  Relational Operator2 : RelationalOperator  Operator===  OutDataTypeStr=boolean  RndMeth=Nearest  InputSameDT=on
  Relational Operator3 : RelationalOperator  Operator===  OutDataTypeStr=boolean  RndMeth=Nearest  InputSameDT=on
  Relational Operator5 : RelationalOperator  Operator===  OutDataTypeStr=boolean  RndMeth=Nearest  InputSameDT=on
  Switch4 : Switch  Criteria=u2 ~= 0  InputSameDT=on
  HLSDEM_TRQDEM_bit19 : Outport
  wires:
  Constant10/1 -> Relational Operator5/2
  Constant3/1 -> Logical Operator9/2
  APP_rUnFlt/1 -> Switch4/1
  APP_r/1 -> Switch4/3
  Relational Operator5/1 -> Switch4/2
  Constant2/1 -> Relational Operator5/1
  Logical Operator9/1 -> HLSDEM_TRQDEM_bit19/1
  Switch4/1 -> Relational Operator1/1
  Constant1/1 -> Relational Operator1/2
  Constant4/1 -> Relational Operator3/2
  Logical Operator6/1 -> Logical Operator9/1
  Relational Operator1/1 -> Logical Operator6/1
  EISGov_numCurrFunc/1 -> Relational Operator2/1, Relational Operator3/1
  Constant5/1 -> Relational Operator2/2
  Relational Operator2/1 -> Logical Operator/2
  Relational Operator3/1 -> Logical Operator/1
  Logical Operator/1 -> Logical Operator6/2

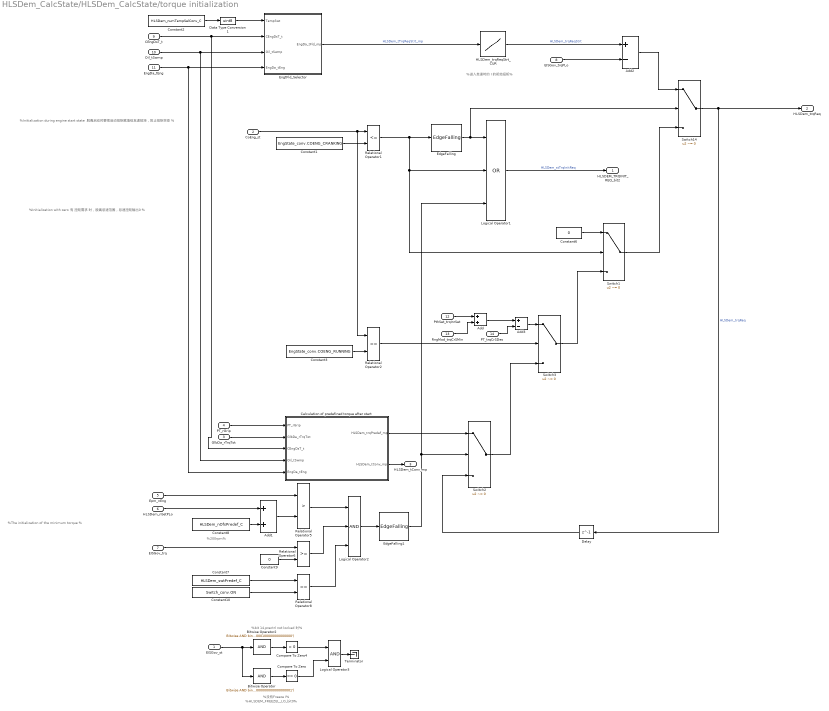
== system HLSDem_CalcState/HLSDem_CalcState/torque initialization ==
  note: %没有Freeze I%
  note: %200rpm%
  note: %进入怠速时的 I 的初始扭矩%
  note: %Initialization with zero
      | 有 扭矩需求 时，脱离怠速范围，怠速扭矩输出0 %
  note: %Initialization during engine start state
      | 脱离启动时要把启动扭矩赋值给怠速扭矩，防止扭矩突变 %
  note: %The initialization of the minimum torque %
  note: %bit 14,prectrl not locked 时%
  note: %HLSDEM_FREEZEL_LO_bit0%
  EISGov_st : Inport
  CoEng_st : Inport  Port=2
  GlbDa_rTrqTot : Inport  Port=3
  PT_rGrip : Inport  Port=4
  Epm_nEng : Inport  Port=5
  HLSDem_nSetPLo : Inport  Port=6
  EISGov_trq : Inport  Port=7
  EISGov_trqPLo : Inport  Port=8
  CEngDsT_t : Inport  Tag=deg  Description=engine coolant temperature after filter  Port=9  OutMin=-200  OutMax=200  OutDataTypeStr=Temp_deg
  Oil_tSwmp : Inport  Tag=deg  Description=Oil temperature in oil sump  Port=10  OutMin=-50  OutMax=200  OutDataTypeStr=Temp_deg
  EngDa_tEng : Inport  Tag=deg  Description=Engine temperature  Port=11  OutMin=-1000  OutMax=1000  OutDataTypeStr=Temp_deg
  PthSet_trqInrSet : Inport  Tag=Nm  Description=Inner torque set value after monitoring limitation  Port=12  OutMin=-3000  OutMax=3276.7  OutDataTypeStr=Trq_Nm
  RngMod_trqCrSMin : Inport  Port=13
  PT_trqCrSDes : Inport  Port=14
  Add : Sum  SaturateOnIntegerOverflow=on
  Add1 : Sum
  Add2 : Sum  Inputs=+-
  Add3 : Sum  Inputs=+-  SaturateOnIntegerOverflow=on
  Bitwise Operator : simulink/Logic and Bit Operations/Bitwise Operator  logicop=AND  UseBitMask=on  BitMask=bin2dec('00000000000000000000000000000001')  BitMaskRealWorld=Stored Integer
  Bitwise Operator2 : simulink/Logic and Bit Operations/Bitwise Operator  logicop=AND  UseBitMask=on  BitMask=bin2dec('00000000000000000100000000000000')  BitMaskRealWorld=Stored Integer
  Calculation of predefined torque after start : Subsystem
  Compare To Zero : simulink/Logic and Bit Operations/Compare To Zero  relop===  OutDataTypeStr=boolean
  Compare To Zero4 : simulink/Logic and Bit Operations/Compare To Zero  relop=>  OutDataTypeStr=boolean
  Constant1 : Constant  Value=EngState_conv.COENG_CRANKING
  Constant10 : Constant  Value=Switch_conv.ON
  Constant2 : Constant  Value=HLSDem_numTempSelConv_C
  Constant3 : Constant  Value=EngState_conv.COENG_RUNNING  OutDataTypeStr=Inherit: Inherit via back propagation
  Constant6 : Constant  Value=0  OutDataTypeStr=Inherit: Inherit via back propagation
  Constant7 : Constant  Value=HLSDem_swtPredef_C
  Constant8 : Constant  Value=HLSDem_nOfsPredef_C
  Constant9 : Constant  Value=0  OutDataTypeStr=Inherit: Inherit via back propagation
  Data Type Conversion1 : DataTypeConversion  OutDataTypeStr=uint8
  Delay : Delay  DelayLength=1  InitialCondition=0
  EdgeFalling : CXLib/EdgeFalling
  EdgeFalling1 : CXLib/EdgeFalling
  EngtFld_Selector : Subsystem
  HLSDem_trqReqStrt_CUR : Lookup_n-D  NumberOfTableDimensions=1  BreakpointsForDimension1=HLSDem_trqReqStrt_CURX  Table=HLSDem_trqReqStrt_CUR  ExtrapMethod=Clip  InternalRulePriority=Speed  OutDataTypeStr=Inherit: Inherit via back propagation  RndMeth=Simplest  SaturateOnIntegerOverflow=on
  Logical Operator1 : Logic  Operator=OR  Inputs=3  OutDataTypeStr=boolean
  Logical Operator2 : Logic  Inputs=3  OutDataTypeStr=boolean
  Logical Operator3 : Logic  OutDataTypeStr=boolean
  Relational Operator1 : RelationalOperator  Operator=<=  OutDataTypeStr=boolean  RndMeth=Nearest  InputSameDT=on
  Relational Operator2 : RelationalOperator  Operator===  OutDataTypeStr=boolean  RndMeth=Nearest  InputSameDT=on
  Relational Operator5 : RelationalOperator  Operator=>  OutDataTypeStr=boolean  RndMeth=Nearest  InputSameDT=on
  Relational Operator6 : RelationalOperator  OutDataTypeStr=boolean  RndMeth=Nearest  InputSameDT=on
  Relational Operator8 : RelationalOperator  Operator===  OutDataTypeStr=boolean  RndMeth=Nearest
  Switch{1..3,14} (4 alike) : Switch  Criteria=u2 ~= 0  InputSameDT=on
  Terminator : Terminator
  HLSDEM_TRQINIT_REQ_bit2 : Outport
  HLSDem_trqReq : Outport  Port=2
  HLSDem_tConv_mp : Outport  Port=3
  wires:
  Delay/1 -> Switch2/3
  Constant6/1 -> Switch1/1
  Switch1/1 -> Switch14/3
  Switch14/1 -> HLSDem_trqReq/1, Delay/1  "HLSDem_trqReq"
  Calculation of predefined torque after start/1(HLSDem_trqPredef_mp) -> Switch2/1
  EngtFld_Selector/1(EngDa_tFld_mp) -> HLSDem_trqReqStrt_CUR/1  "HLSDem_tTrqReqStrt_mp"
  Add1/1 -> Relational Operator5/2
  Constant8/1 -> Add1/2
  Constant9/1 -> Relational Operator6/2
  Constant7/1 -> Relational Operator8/1
  Constant10/1 -> Relational Operator8/2
  Relational Operator5/1 -> Logical Operator2/1
  HLSDem_nSetPLo/1 -> Add1/1
  EISGov_trq/1 -> Relational Operator6/1
  Compare To Zero4/1 -> Logical Operator3/1
  Bitwise Operator/1 -> Compare To Zero/1
  Compare To Zero/1 -> Logical Operator3/2
  Add2/1 -> Switch14/1
  EISGov_trqPLo/1 -> Add2/2
  EdgeFalling/1 -> Switch14/2, Logical Operator1/1
  Logical Operator1/1 -> HLSDEM_TRQINIT_REQ_bit2/1  "HLSDem_stTrqInitReq"
  Bitwise Operator2/1 -> Compare To Zero4/1
  Relational Operator6/1 -> Logical Operator2/2
  GlbDa_rTrqTot/1 -> Calculation of predefined torque after start/2(GlbDa_rTrqTot)
  PT_rGrip/1 -> Calculation of predefined torque after start/1(PT_rGrip)
  HLSDem_trqReqStrt_CUR/1 -> Add2/1  "HLSDem_trqReqStrt"
  EISGov_st/1 -> Bitwise Operator/1, Bitwise Operator2/1
  Constant1/1 -> Relational Operator1/2
  Relational Operator1/1 -> Switch1/2, Logical Operator1/2, EdgeFalling/1
  Epm_nEng/1 -> Relational Operator5/1
  Relational Operator8/1 -> Logical Operator2/3
  Constant2/1 -> Data Type Conversion1/1
  Data Type Conversion1/1 -> EngtFld_Selector/1(TempSwt)
  CEngDsT_t/1 -> EngtFld_Selector/2(CEngDsT_t), Calculation of predefined torque after start/3(CEngDsT_t)
  Oil_tSwmp/1 -> EngtFld_Selector/3(Oil_tSwmp), Calculation of predefined torque after start/4(Oil_tSwmp)
  EngDa_tEng/1 -> EngtFld_Selector/4(EngDa_tEng), Calculation of predefined torque after start/5(EngDa_tEng)
  Logical Operator3/1 -> Terminator/1
  CoEng_st/1 -> Relational Operator2/1, Relational Operator1/1
  Constant3/1 -> Relational Operator2/2
  Relational Operator2/1 -> Switch3/2
  Switch3/1 -> Switch1/3
  Switch2/1 -> Switch3/3
  PthSet_trqInrSet/1 -> Add/1
  RngMod_trqCrSMin/1 -> Add/2
  Add/1 -> Add3/1
  Add3/1 -> Switch3/1
  PT_trqCrSDes/1 -> Add3/2
  Calculation of predefined torque after start/2(HLSDem_tConv_mp) -> HLSDem_tConv_mp/1
  Logical Operator2/1 -> EdgeFalling1/1
  EdgeFalling1/1 -> Logical Operator1/3, Switch2/2

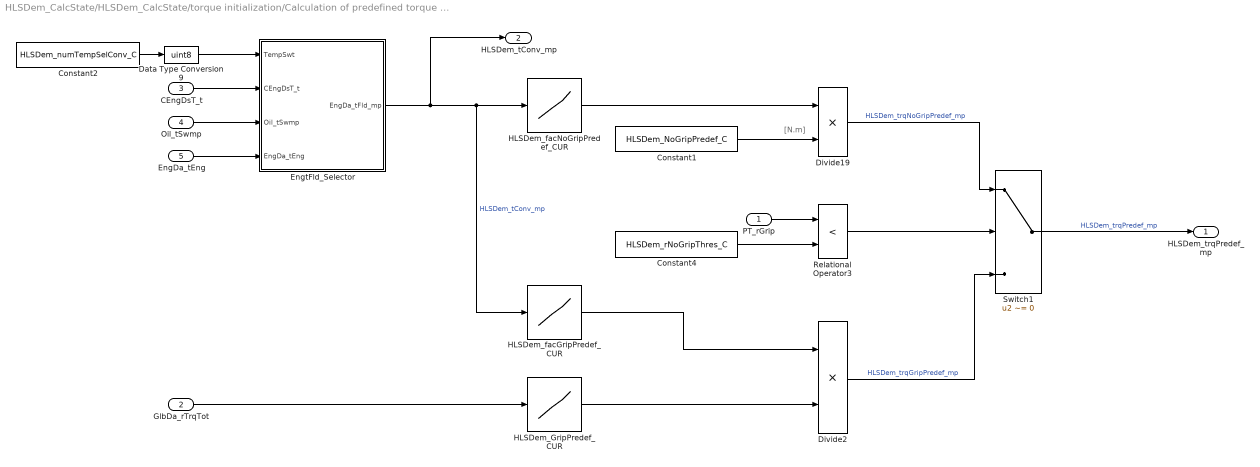
== system HLSDem_CalcState/HLSDem_CalcState/torque initialization/Calculation of predefined torque after start ==
  note: [N.m]
  PT_rGrip : Inport
  GlbDa_rTrqTot : Inport  Port=2
  CEngDsT_t : Inport  Tag=deg  Description=engine coolant temperature after filter  Port=3  OutMin=-200  OutMax=200  OutDataTypeStr=Temp_deg
  Oil_tSwmp : Inport  Tag=deg  Description=Oil temperature in oil sump  Port=4  OutMin=-50  OutMax=200  OutDataTypeStr=Temp_deg
  EngDa_tEng : Inport  Tag=deg  Description=Engine temperature  Port=5  OutMin=-1000  OutMax=1000  OutDataTypeStr=Temp_deg
  Constant1 : Constant  Value=HLSDem_NoGripPredef_C
  Constant2 : Constant  Value=HLSDem_numTempSelConv_C
  Constant4 : Constant  Value=HLSDem_rNoGripThres_C
  Data Type Conversion9 : DataTypeConversion  OutDataTypeStr=uint8
  Divide19 : Product  Inputs=**  OutDataTypeStr=Trq_Nm  RndMeth=Round  SaturateOnIntegerOverflow=on
  Divide2 : Product  Inputs=**  OutDataTypeStr=Trq_Nm  SaturateOnIntegerOverflow=on
  EngtFld_Selector : Subsystem
  HLSDem_GripPredef_CUR : Lookup_n-D  NumberOfTableDimensions=1  BreakpointsForDimension1=HLSDem_GripPredef_CURX  Table=HLSDem_GripPredef_CUR  ExtrapMethod=Clip  InternalRulePriority=Speed  OutDataTypeStr=Inherit: Inherit via back propagation  RndMeth=Simplest  SaturateOnIntegerOverflow=on
  HLSDem_facGripPredef_CUR : Lookup_n-D  NumberOfTableDimensions=1  BreakpointsForDimension1=HLSDem_facGripPredef_CURX  Table=HLSDem_facGripPredef_CUR  ExtrapMethod=Clip  InternalRulePriority=Speed  OutDataTypeStr=Inherit: Inherit via back propagation  RndMeth=Simplest  SaturateOnIntegerOverflow=on
  HLSDem_facNoGripPredef_CUR : Lookup_n-D  NumberOfTableDimensions=1  BreakpointsForDimension1=HLSDem_facNoGripPredef_CURX  Table=HLSDem_facNoGripPredef_CUR  ExtrapMethod=Clip  InternalRulePriority=Speed  OutDataTypeStr=Inherit: Inherit via back propagation  RndMeth=Simplest  SaturateOnIntegerOverflow=on
  Relational Operator3 : RelationalOperator  Operator=<  OutDataTypeStr=boolean  RndMeth=Nearest  InputSameDT=on
  Switch1 : Switch  Criteria=u2 ~= 0  InputSameDT=on
  HLSDem_trqPredef_mp : Outport
  HLSDem_tConv_mp : Outport  Port=2
  wires:
  Constant1/1 -> Divide19/2
  HLSDem_facNoGripPredef_CUR/1 -> Divide19/1
  Divide2/1 -> Switch1/3  "HLSDem_trqGripPredef_mp"
  HLSDem_facGripPredef_CUR/1 -> Divide2/1
  PT_rGrip/1 -> Relational Operator3/1
  Relational Operator3/1 -> Switch1/2
  EngtFld_Selector/1(EngDa_tFld_mp) -> HLSDem_tConv_mp/1, HLSDem_facGripPredef_CUR/1, HLSDem_facNoGripPredef_CUR/1  "HLSDem_tConv_mp"
  Divide19/1 -> Switch1/1  "HLSDem_trqNoGripPredef_mp"
  Constant2/1 -> Data Type Conversion9/1
  Switch1/1 -> HLSDem_trqPredef_mp/1  "HLSDem_trqPredef_mp"
  GlbDa_rTrqTot/1 -> HLSDem_GripPredef_CUR/1
  Constant4/1 -> Relational Operator3/2
  HLSDem_GripPredef_CUR/1 -> Divide2/2
  Data Type Conversion9/1 -> EngtFld_Selector/1(TempSwt)
  CEngDsT_t/1 -> EngtFld_Selector/2(CEngDsT_t)
  Oil_tSwmp/1 -> EngtFld_Selector/3(Oil_tSwmp)
  EngDa_tEng/1 -> EngtFld_Selector/4(EngDa_tEng)

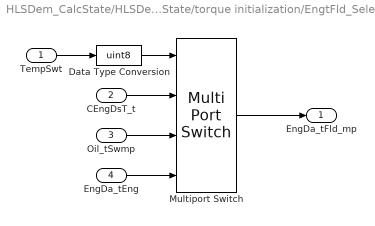
== system HLSDem_CalcState/HLSDem_CalcState/torque initialization/EngtFld_Selector ==
  TempSwt : Inport
  CEngDsT_t : Inport  Tag=deg  Description=engine coolant temperature after filter  Port=2
  Oil_tSwmp : Inport  Tag=deg  Description=Oil temperature in oil sump  Port=3
  EngDa_tEng : Inport  Tag=deg  Description=Engine temperature  Port=4
  Data Type Conversion : DataTypeConversion  OutDataTypeStr=uint8
  Multiport Switch : MultiPortSwitch  DataPortOrder=Zero-based contiguous
  EngDa_tFld_mp : Outport  Tag=deg  Description=Engine temperature field
  wires:
  CEngDsT_t/1 -> Multiport Switch/2
  Multiport Switch/1 -> EngDa_tFld_mp/1
  EngDa_tEng/1 -> Multiport Switch/4
  Oil_tSwmp/1 -> Multiport Switch/3
  Data Type Conversion/1 -> Multiport Switch/1
  TempSwt/1 -> Data Type Conversion/1

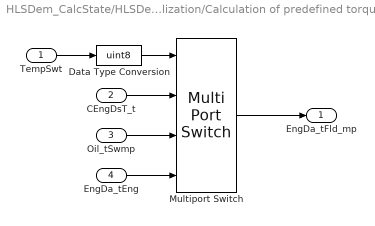
== system HLSDem_CalcState/HLSDem_CalcState/torque initialization/Calculation of predefined torque after start/EngtFld_Selector ==
  TempSwt : Inport
  CEngDsT_t : Inport  Tag=deg  Description=engine coolant temperature after filter  Port=2
  Oil_tSwmp : Inport  Tag=deg  Description=Oil temperature in oil sump  Port=3
  EngDa_tEng : Inport  Tag=deg  Description=Engine temperature  Port=4
  Data Type Conversion : DataTypeConversion  OutDataTypeStr=uint8
  Multiport Switch : MultiPortSwitch  DataPortOrder=Zero-based contiguous
  EngDa_tFld_mp : Outport  Tag=deg  Description=Engine temperature field
  wires:
  CEngDsT_t/1 -> Multiport Switch/2
  Multiport Switch/1 -> EngDa_tFld_mp/1
  EngDa_tEng/1 -> Multiport Switch/4
  Oil_tSwmp/1 -> Multiport Switch/3
  Data Type Conversion/1 -> Multiport Switch/1
  TempSwt/1 -> Data Type Conversion/1

== stateflow chart HLSDem_CalcState/DT1 activation/Chart ==
  note: %clear bit 8.9.10,11%
  state EISGov_STD_INACTIVE
    during:EISGov_st_out=EISGov_st & 0xfff0ff;
  note: %set bit 10%
  state EISGov_STDFALL_PREP
    during:EISGov_st_out=(EISGov_st & 0xfff0ff) | 0x000400;
  state EISGov_STDFALL_ACTIVE
    during:EISGov_st_out=EISGov_st | 0x000800;
  note: %set bit 11%
  (default) -> EISGov_STD_INACTIVE
  EISGov_STD_INACTIVE -> EISGov_STDFALL_PREP : [((EISGov_nSetpointLo+EISGov_nOfsPreCtlPrepFallCurr_mp)<Epm_nEng) &&...
      | (CoEng_st >= EngState_conv.COENG_RUNNING)]
  EISGov_STDFALL_PREP -> EISGov_STD_INACTIVE [order 1] : [(EISGov_nSetpointLo + EISGov_nOfsPreCtlINActvFallCurr_mp) >=Epm_nEng]
  EISGov_STDFALL_ACTIVE -> EISGov_STD_INACTIVE [order 2] : [(EISGov_nSetpointLo + EISGov_nOfsPreCtlINActvFallCurr_mp) >=Epm_nEng]
  EISGov_STDFALL_PREP -> EISGov_STDFALL_ACTIVE [order 2] : [(EISGov_nSetpointLo+...
      | EISGov_nOfsPreCtlActvFallCurr_mp) > Epm_nEng]
  EISGov_STDFALL_ACTIVE -> EISGov_STDFALL_PREP [order 1] : [(EISGov_nSetpointLo+...
      | EISGov_nOfsPreCtlActvFallCurr_mp) < Epm_nEng]
  data: Epm_nEng input; CoEng_st input; EISGov_st input; EISGov_nSetpointLo input; EISGov_nOfsPreCtlPrepFallCurr_mp input; EISGov_nOfsPreCtlActvFallCurr_mp input; EISGov_st_out output; EISGov_nOfsPreCtlINActvFallCurr_mp input
